simulink model "exampleModel_bus_axi_lcls2"  (R2017b)
settings: Solver=VariableStepAuto  StartTime=0.0  StopTime=10e-5  RelTol=1e-3
PreLoadFcn:
  | setup
values from neighbouring files (symbols this model uses):
  axiClk = 156.25e6    (= 156250000)    [setup.m]    (also in setup_exampleModel_bus_axi_simulink.m; setup_exampleModel_bus_axi_simulink_lcls2.m; setup_lcls2_pcav.m; sysgen_signal.m)
  cav1p1_addr = 204    [setup_exampleModel_bus_axi_simulink.m]    (also in setup_exampleModel_bus_axi_simulink_lcls2.m; setup_lcls2_pcav.m; sysgen_signal.m)
  cav1p2_addr = cav1p1_addr * 2    (= 408)    [setup_exampleModel_bus_axi_simulink.m]    (also in setup_exampleModel_bus_axi_simulink_lcls2.m; setup_lcls2_pcav.m; sysgen_signal.m)
  cav2p1_addr = cav1p1_addr * 3    (= 612)    [setup_exampleModel_bus_axi_simulink.m]    (also in setup_exampleModel_bus_axi_simulink_lcls2.m; setup_lcls2_pcav.m; sysgen_signal.m)
  cav2p2_addr = cav1p1_addr * 4    (= 816)    [setup_exampleModel_bus_axi_simulink.m]    (also in setup_exampleModel_bus_axi_simulink_lcls2.m; setup_lcls2_pcav.m; sysgen_signal.m)
  Fadc = Fs/interleavedChannels    (= 29750000)    [setup.m]    (also in setup_exampleModel_bus_axi_simulink.m = 357000000; setup_exampleModel_bus_axi_simulink_lcls2.m = 351000000; setup_lcls2_pcav.m = 357000000; sysgen_signal.m = 357000000)
  Fproc = 204e6    (= 204000000)    [setup_exampleModel_bus_axi_simulink.m]    (also in setup_exampleModel_bus_axi_simulink_lcls2.m = 200571400; setup_lcls2_pcav.m; sysgen_signal.m)
  Fsig = Fproc/12    (= 17000000)    [setup_exampleModel_bus_axi_simulink.m]    (also in setup_exampleModel_bus_axi_simulink_lcls2.m = 16714283.3333; setup_lcls2_pcav.m)
  Tadc = 1/fadc    (= 2.80112044818e-09)    [cavity_signal.m]    (also in setup_exampleModel_bus_axi_simulink.m; setup_exampleModel_bus_axi_simulink_lcls2.m = 2.849002849e-09; setup_lcls2_pcav.m; setup_pcav_simulink.m)
undefined symbols (not defined in the file or in its folder): AXI4, Lite
libraries: xbsIndex_r4 x2055, llrf_lib x10, simulink x1
(part 1 of 12)
settings Model: Creator=mdewart  LastModifiedBy=isils

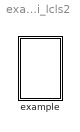
== system exampleModel_bus_axi_lcls2 ==
  example : Subsystem

== system exampleModel_bus_axi_lcls2/example ==
  note: Cav1
  note: use this system generator block to build
  note: Cav1 port 1 2
  note: Reference
  note: RF Ref
  note: Cav2
  note: Cav2 port 1 2
  " System Generator" : xbsIndex_r4/ System Generator  Tag=genX  xilinxfamily=kintexu  part=xcku040  speed=-2-e  package=ffva1156  synthesis_tool=Vivado  clock_wrapper=Clock Enables  directory=./netlist  proj_type=Vivado  Synth_file=Vivado Synthesis Defaults  Impl_file=Vivado Implementation Defaults  testbench=off  simulink_period=2/Fadc  sysclk_period=2e9/(Fadc)  dcm_input_clock_period=10  incr_netlist=off  trim_vbits=Everywhere in SubSystem  dbl_ovrd=According to Block Masks  core_generation=According to Block Masks  run_coregen=off  deprecated_control=off  eval_field=0  block_type=sysgen
  Subsystem : Subsystem
  Subsystem2 : Subsystem
  Subsystem3 : Subsystem
  Subsystem4 : Subsystem
  Subsystem5 : Subsystem
  Subsystem7 : Subsystem
  axi_lite : Subsystem
  dsp : Subsystem
  wires:
  Subsystem/2(P2) -> axi_lite/3(In3)
  Subsystem/1(P1) -> axi_lite/2(In2)
  Subsystem3/1(Out1) -> axi_lite/1(In1)
  axi_lite/2(Out2) -> Subsystem2/1(In1)
  axi_lite/1(Out1) -> Subsystem4/1(In1)
  Subsystem5/1(P1) -> axi_lite/4(In4)
  Subsystem5/2(P2) -> axi_lite/5(In5)
  axi_lite/3(Out3) -> Subsystem7/1(In1)

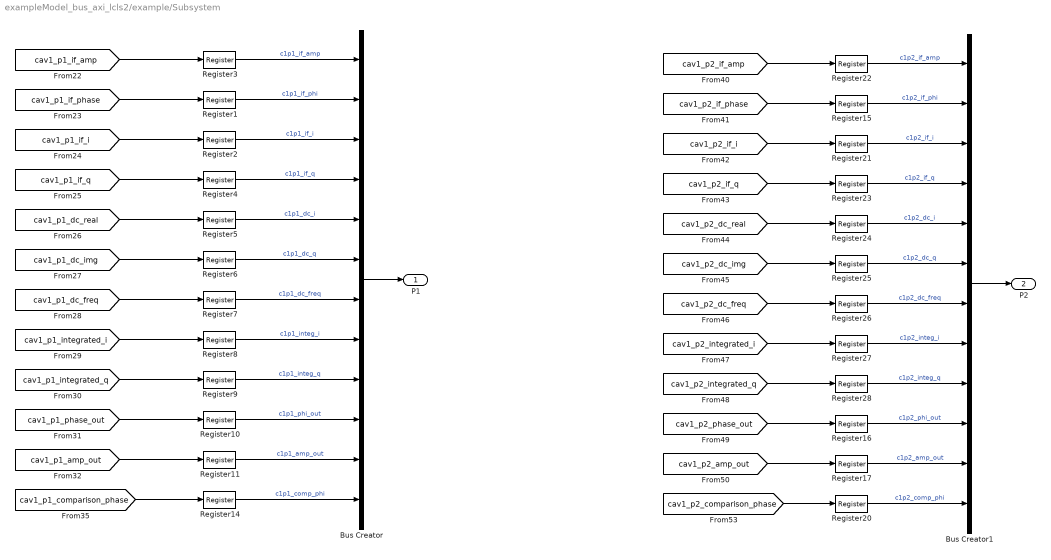
== system exampleModel_bus_axi_lcls2/example/Subsystem ==
  Bus Creator : BusCreator  Inputs=12
  Bus Creator1 : BusCreator  Inputs=12
  Register{1..11,14..17,20..28} (24 alike) : xbsIndex_r4/Register  init=0  rst=off  en=off  dbl_ovrd=off  block_type=register
  P1 : Outport
  P2 : Outport  Port=2
  wires:
  Register1/1 -> Bus Creator/2  "c1p1_if_phi"
  Register9/1 -> Bus Creator/9  "c1p1_integ_q"
  Register14/1 -> Bus Creator/12  "c1p1_comp_phi"
  [cav1_p1_integrated_i] -> Register8/1
  [cav1_p1_phase_out] -> Register10/1
  Register10/1 -> Bus Creator/10  "c1p1_phi_out"
  [cav1_p1_amp_out] -> Register11/1
  Register2/1 -> Bus Creator/3  "c1p1_if_i"
  Register4/1 -> Bus Creator/4  "c1p1_if_q"
  Register6/1 -> Bus Creator/6  "c1p1_dc_q"
  Register11/1 -> Bus Creator/11  "c1p1_amp_out"
  [cav1_p1_dc_img] -> Register6/1
  Register7/1 -> Bus Creator/7  "c1p1_dc_freq"
  Register8/1 -> Bus Creator/8  "c1p1_integ_i"
  [cav1_p1_if_amp] -> Register3/1
  [cav1_p1_if_phase] -> Register1/1
  [cav1_p1_if_i] -> Register2/1
  [cav1_p1_if_q] -> Register4/1
  [cav1_p1_dc_real] -> Register5/1
  [cav1_p1_integrated_q] -> Register9/1
  [cav1_p1_dc_freq] -> Register7/1
  [cav1_p1_comparison_phase] -> Register14/1
  Register3/1 -> Bus Creator/1  "c1p1_if_amp"
  Register5/1 -> Bus Creator/5  "c1p1_dc_i"
  Bus Creator/1 -> P1/1
  [cav1_p2_if_q] -> Register23/1
  Register21/1 -> Bus Creator1/3  "c1p2_if_i"
  Register20/1 -> Bus Creator1/12  "c1p2_comp_phi"
  Register24/1 -> Bus Creator1/5  "c1p2_dc_i"
  Register17/1 -> Bus Creator1/11  "c1p2_amp_out"
  Register25/1 -> Bus Creator1/6  "c1p2_dc_q"
  Register15/1 -> Bus Creator1/2  "c1p2_if_phi"
  Register23/1 -> Bus Creator1/4  "c1p2_if_q"
  [cav1_p2_phase_out] -> Register16/1
  Register16/1 -> Bus Creator1/10  "c1p2_phi_out"
  [cav1_p2_if_phase] -> Register15/1
  Register26/1 -> Bus Creator1/7  "c1p2_dc_freq"
  Register22/1 -> Bus Creator1/1  "c1p2_if_amp"
  [cav1_p2_comparison_phase] -> Register20/1
  Bus Creator1/1 -> P2/1
  [cav1_p2_dc_real] -> Register24/1
  [cav1_p2_dc_freq] -> Register26/1
  [cav1_p2_integrated_q] -> Register28/1
  [cav1_p2_if_amp] -> Register22/1
  Register28/1 -> Bus Creator1/9  "c1p2_integ_q"
  [cav1_p2_dc_img] -> Register25/1
  [cav1_p2_amp_out] -> Register17/1
  Register27/1 -> Bus Creator1/8  "c1p2_integ_i"
  [cav1_p2_if_i] -> Register21/1
  [cav1_p2_integrated_i] -> Register27/1

== system exampleModel_bus_axi_lcls2/example/Subsystem2 ==
  In1 : Inport
  Bus Selector : BusSelector  OutputSignals=c1p1_chan_sel,c1p2_chan_sel,c1p1_win_start,c1p1_win_stop,c1p2_win_start,c1p2_win_stop,c1_nco_reset,c1_nco_phi,c1p1_cal_coeff,c1p2_cal_coeff,c1_freq_win_start,c1_freq_win_stop,ca_reg_latch_pt
  Register{1..5,29..31,33,35..36} (11 alike) : xbsIndex_r4/Register  init=0  rst=off  en=off  dbl_ovrd=off  block_type=register
  Register32 : xbsIndex_r4/Register  init=100  rst=off  en=off  dbl_ovrd=off  block_type=register
  Register34 : xbsIndex_r4/Register  init=100  rst=off  en=off  dbl_ovrd=off  block_type=register
  tag scope: cav1_f_window_start=global, cav1_f_window_stop=global, cav1_nco_phase_adj=global, cav1_nco_phase_reset=global, cav1_p1_cal_coef=global, cav1_p1_chan_sel=global, cav1_p1_window_start=global, cav1_p1_window_stop=global, cav1_p2_cal_coef=global, cav1_p2_chan_sel=global, cav1_p2_window_start=global, cav1_p2_window_stop=global, cav1_reg_latch_pt=global
  wires:
  Register30/1 -> [cav1_p2_chan_sel]
  Register34/1 -> [cav1_p2_window_stop]
  Register35/1 -> [cav1_nco_phase_reset]
  Register29/1 -> [cav1_p1_chan_sel]
  Register32/1 -> [cav1_p1_window_stop]
  Register36/1 -> [cav1_nco_phase_adj]
  Register33/1 -> [cav1_p2_window_start]
  Register31/1 -> [cav1_p1_window_start]
  In1/1 -> Bus Selector/1
  Bus Selector/1 -> Register29/1  "<c1p1_chan_sel>"
  Bus Selector/2 -> Register30/1  "<c1p2_chan_sel>"
  Bus Selector/3 -> Register31/1  "<c1p1_win_start>"
  Bus Selector/4 -> Register32/1  "<c1p1_win_stop>"
  Bus Selector/5 -> Register33/1  "<c1p2_win_start>"
  Bus Selector/6 -> Register34/1  "<c1p2_win_stop>"
  Bus Selector/7 -> Register35/1  "<c1_nco_reset>"
  Bus Selector/8 -> Register36/1  "<c1_nco_phi>"
  Bus Selector/9 -> Register1/1  "<c1p1_cal_coeff>"
  Bus Selector/10 -> Register2/1  "<c1p2_cal_coeff>"
  Register1/1 -> [cav1_p1_cal_coef]
  Register2/1 -> [cav1_p2_cal_coef]
  Register3/1 -> [cav1_f_window_start]
  Register4/1 -> [cav1_f_window_stop]
  Bus Selector/12 -> Register4/1  "<c1_freq_win_stop>"
  Bus Selector/11 -> Register3/1  "<c1_freq_win_start>"
  Register5/1 -> [cav1_reg_latch_pt]
  Bus Selector/13 -> Register5/1  "<ca_reg_latch_pt>"

== system exampleModel_bus_axi_lcls2/example/Subsystem3 ==
  Bus Creator : BusCreator  Inputs=4
  Register{1..4} (4 alike) : xbsIndex_r4/Register  init=0  rst=off  en=off  dbl_ovrd=off  block_type=register
  Out1 : Outport
  wires:
  Register4/1 -> Bus Creator/4  "ref_q"
  Register2/1 -> Bus Creator/3  "ref_i"
  [ref_q_phase] -> Register1/1
  [ref_i_reg] -> Register2/1
  [ref_i_amp] -> Register3/1
  Register3/1 -> Bus Creator/1  "ref_amp"
  Register1/1 -> Bus Creator/2  "ref_phi"
  [ref_q_reg] -> Register4/1
  Bus Creator/1 -> Out1/1

== system exampleModel_bus_axi_lcls2/example/Subsystem4 ==
  In1 : Inport
  Bus Selector : BusSelector  OutputSignals=ref_chan_sel,wfdata_0_sel,wfdata_1_sel,wfdata_2_sel,wfdata_3_sel,wfdata_4_sel,wfdata_5_sel,wfdata_6_sel,wfdata_7_sel
  Register{1..9} (9 alike) : xbsIndex_r4/Register  init=0  rst=off  en=off  dbl_ovrd=off  block_type=register
  tag scope: rf_ref_chan_sel=global, wfdata_0_sel=global, wfdata_1_sel=global, wfdata_2_sel=global, wfdata_3_sel=global, wfdata_4_sel=global, wfdata_5_sel=global, wfdata_6_sel=global, wfdata_7_sel=global
  wires:
  Register2/1 -> [rf_ref_chan_sel]
  Bus Selector/1 -> Register2/1  "<ref_chan_sel>"
  In1/1 -> Bus Selector/1
  Bus Selector/2 -> Register1/1  "<wfdata_0_sel>"
  Bus Selector/3 -> Register3/1  "<wfdata_1_sel>"
  Bus Selector/4 -> Register4/1  "<wfdata_2_sel>"
  Bus Selector/5 -> Register5/1  "<wfdata_3_sel>"
  Bus Selector/6 -> Register6/1  "<wfdata_4_sel>"
  Bus Selector/7 -> Register7/1  "<wfdata_5_sel>"
  Bus Selector/8 -> Register8/1  "<wfdata_6_sel>"
  Bus Selector/9 -> Register9/1  "<wfdata_7_sel>"
  Register9/1 -> [wfdata_7_sel]
  Register8/1 -> [wfdata_6_sel]
  Register7/1 -> [wfdata_5_sel]
  Register6/1 -> [wfdata_4_sel]
  Register5/1 -> [wfdata_3_sel]
  Register4/1 -> [wfdata_2_sel]
  Register3/1 -> [wfdata_1_sel]
  Register1/1 -> [wfdata_0_sel]

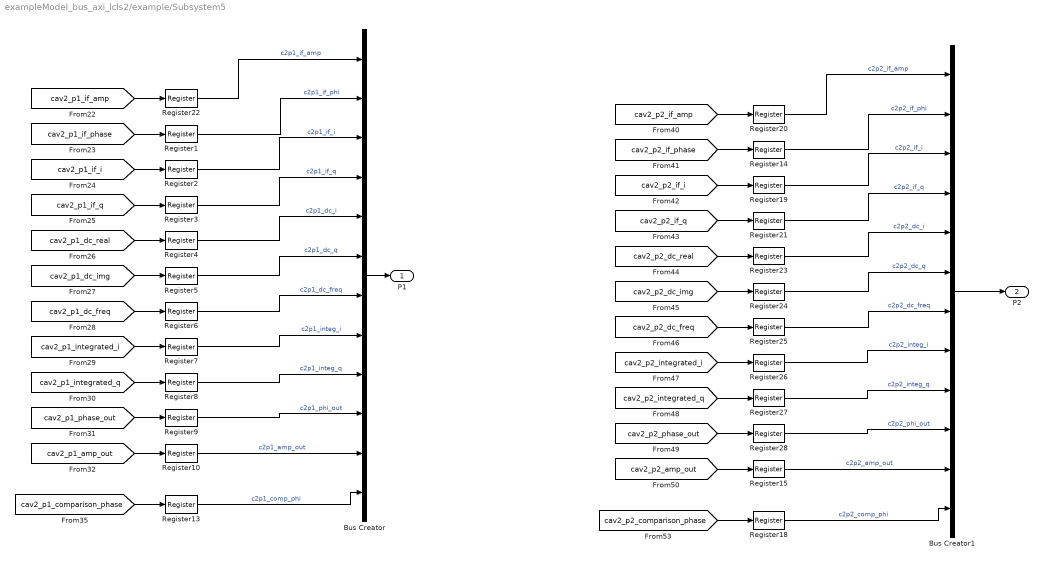
== system exampleModel_bus_axi_lcls2/example/Subsystem5 ==
  Bus Creator : BusCreator  Inputs=12
  Bus Creator1 : BusCreator  Inputs=12
  Register{1..10,13..15,18..28} (24 alike) : xbsIndex_r4/Register  init=0  rst=off  en=off  dbl_ovrd=off  block_type=register
  P1 : Outport
  P2 : Outport  Port=2
  wires:
  Register9/1 -> Bus Creator/10  "c2p1_phi_out"
  Register13/1 -> Bus Creator/12  "c2p1_comp_phi"
  Register2/1 -> Bus Creator/3  "c2p1_if_i"
  Register6/1 -> Bus Creator/7  "c2p1_dc_freq"
  Register10/1 -> Bus Creator/11  "c2p1_amp_out"
  Register7/1 -> Bus Creator/8  "c2p1_integ_i"
  Register3/1 -> Bus Creator/4  "c2p1_if_q"
  Register1/1 -> Bus Creator/2  "c2p1_if_phi"
  Register4/1 -> Bus Creator/5  "c2p1_dc_i"
  Register5/1 -> Bus Creator/6  "c2p1_dc_q"
  Register8/1 -> Bus Creator/9  "c2p1_integ_q"
  Bus Creator/1 -> P1/1
  Register22/1 -> Bus Creator/1  "c2p1_if_amp"
  [cav2_p1_if_amp] -> Register22/1
  [cav2_p1_comparison_phase] -> Register13/1
  [cav2_p1_amp_out] -> Register10/1
  [cav2_p1_phase_out] -> Register9/1
  [cav2_p1_integrated_q] -> Register8/1
  [cav2_p1_integrated_i] -> Register7/1
  [cav2_p1_dc_freq] -> Register6/1
  [cav2_p1_dc_img] -> Register5/1
  [cav2_p1_dc_real] -> Register4/1
  [cav2_p1_if_q] -> Register3/1
  [cav2_p1_if_i] -> Register2/1
  [cav2_p1_if_phase] -> Register1/1
  [cav2_p2_comparison_phase] -> Register18/1
  Bus Creator1/1 -> P2/1
  [cav2_p2_if_phase] -> Register14/1
  Register26/1 -> Bus Creator1/8  "c2p2_integ_i"
  [cav2_p2_dc_real] -> Register23/1
  Register19/1 -> Bus Creator1/3  "c2p2_if_i"
  [cav2_p2_integrated_q] -> Register27/1
  Register28/1 -> Bus Creator1/10  "c2p2_phi_out"
  Register23/1 -> Bus Creator1/5  "c2p2_dc_i"
  Register27/1 -> Bus Creator1/9  "c2p2_integ_q"
  [cav2_p2_dc_img] -> Register24/1
  [cav2_p2_phase_out] -> Register28/1
  Register25/1 -> Bus Creator1/7  "c2p2_dc_freq"
  Register15/1 -> Bus Creator1/11  "c2p2_amp_out"
  [cav2_p2_integrated_i] -> Register26/1
  Register21/1 -> Bus Creator1/4  "c2p2_if_q"
  [cav2_p2_if_amp] -> Register20/1
  [cav2_p2_amp_out] -> Register15/1
  [cav2_p2_if_q] -> Register21/1
  Register20/1 -> Bus Creator1/1  "c2p2_if_amp"
  [cav2_p2_dc_freq] -> Register25/1
  Register18/1 -> Bus Creator1/12  "c2p2_comp_phi"
  Register14/1 -> Bus Creator1/2  "c2p2_if_phi"
  [cav2_p2_if_i] -> Register19/1
  Register24/1 -> Bus Creator1/6  "c2p2_dc_q"

== system exampleModel_bus_axi_lcls2/example/Subsystem7 ==
  In1 : Inport
  Bus Selector : BusSelector  OutputSignals=c2p1_chan_sel,c2p2_chan_sel,c2p1_win_start,c2p1_win_stop,c2p2_win_start,c2p2_win_stop,c2_nco_reset,c2_nco_phi,c2p1_cal_coeff,c2p2_cal_coeff,c2_freq_win_start,c2_freq_win_stop,ca_reg_latch_pt
  Register{1..5,29..36} (13 alike) : xbsIndex_r4/Register  init=0  rst=off  en=off  dbl_ovrd=off  block_type=register
  tag scope: cav2_f_window_start=global, cav2_f_window_stop=global, cav2_nco_phase_adj=global, cav2_nco_phase_reset=global, cav2_p1_cal_coef=global, cav2_p1_chan_sel=global, cav2_p1_window_start=global, cav2_p1_window_stop=global, cav2_p2_cal_coef=global, cav2_p2_chan_sel=global, cav2_p2_window_start=global, cav2_p2_window_stop=global, cav2_reg_latch_pt=global
  wires:
  Bus Selector/8 -> Register36/1  "<c2_nco_phi>"
  Bus Selector/7 -> Register35/1  "<c2_nco_reset>"
  Bus Selector/6 -> Register34/1  "<c2p2_win_stop>"
  Bus Selector/5 -> Register33/1  "<c2p2_win_start>"
  Bus Selector/4 -> Register32/1  "<c2p1_win_stop>"
  Bus Selector/3 -> Register31/1  "<c2p1_win_start>"
  Bus Selector/2 -> Register30/1  "<c2p2_chan_sel>"
  Bus Selector/1 -> Register29/1  "<c2p1_chan_sel>"
  In1/1 -> Bus Selector/1
  Register31/1 -> [cav2_p1_window_start]
  Register33/1 -> [cav2_p2_window_start]
  Register36/1 -> [cav2_nco_phase_adj]
  Register32/1 -> [cav2_p1_window_stop]
  Register29/1 -> [cav2_p1_chan_sel]
  Register35/1 -> [cav2_nco_phase_reset]
  Register34/1 -> [cav2_p2_window_stop]
  Register30/1 -> [cav2_p2_chan_sel]
  Register1/1 -> [cav2_p1_cal_coef]
  Register2/1 -> [cav2_p2_cal_coef]
  Bus Selector/9 -> Register1/1  "<c2p1_cal_coeff>"
  Bus Selector/10 -> Register2/1  "<c2p2_cal_coeff>"
  Register5/1 -> [cav2_reg_latch_pt]
  Register3/1 -> [cav2_f_window_start]
  Register4/1 -> [cav2_f_window_stop]
  Bus Selector/11 -> Register3/1  "<c2_freq_win_start>"
  Bus Selector/12 -> Register4/1  "<c2_freq_win_stop>"
  Bus Selector/13 -> Register5/1  "<ca_reg_latch_pt>"
